simulink model "cs_robot"  (R2017b)
settings: Solver=FixedStepDiscrete  StartTime=0.0  StopTime=2  RelTol=1e-3  EnableMultiTasking=on
PreLoadFcn:
  | Ts=1e-6;
InitFcn:
  | Ts=1e-6;
undefined symbols (not defined in the file): DiscIntNeverNeededParam
libraries: powerlib x5, electricdrivelib x4
Description:
  | Copyright 2008-2017 The MathWorks, Inc.
settings Model: ExtModeAutoUpdateStatusClock=off  Creator=MathWorks  LastModifiedBy=Rafa
settings SolverCC: InsertRTBMode=Auto
settings DataIOCC: LimitDataPoints=on  SaveFormat=Array  SignalLoggingSaveFormat=ModelDataLogs  SignalLoggingName=sigsOut
settings OptimizationCC: ExpressionDepthLimit=2147483647  InitFltsAndDblsToZero=on  LifeSpan=inf
settings DebuggingCC: SaveWithParameterizedLinksMsg=none  UnderspecifiedInitializationDetection=Classic  MergeDetectMultiDrivingBlocksExec=none  CheckExecutionContextPreStartOutputMsg=on  CheckExecutionContextRuntimeOutputMsg=on  SignalResolutionControl=TryResolveAllWithWarning  MultiTaskDSMMsg=warning  MultiTaskCondExecSysMsg=none  FcnCallInpInsideContextMsg=warning  AllowSymbolicDim=off  StateNameClashWarn=warning  SFUnexpectedBacktrackingDiag=warning  SFNoUnconditionalDefaultTransitionDiag=warning  SFExecutionAtInitializationDiag=none
settings HardwareCC: ProdBitPerPointer=32  ProdBitPerSizeT=32  ProdBitPerPtrDiffT=32  ProdLargestAtomicFloat=None  ProdIntDivRoundTo=Undefined  ProdEndianess=Unspecified  ProdWordSize=32  ProdHWDeviceType=32-bit Generic  TargetBitPerPointer=64  TargetBitPerSizeT=64  TargetBitPerPtrDiffT=64  TargetLongLongMode=on  TargetIntDivRoundTo=Zero  TargetEndianess=LittleEndian  TargetWordSize=64  TargetHWDeviceType=MATLAB Host  ProdEqTarget=off
settings ModelReferenceCC: PropagateSignalLabelsOutOfModel=off
settings CodeAppCC: StateflowObjectComments=on
settings GRTTargetCC: TargetFcnLib=ansi_tfl_tmw.mat  TargetLangStandard=C89/C90 (ANSI)  GeneratePreprocessorConditionals=Disable all  CombineOutputUpdateFcns=off  GRTInterface=on
settings ConfigComp: CovMetricSettings=dw  CovHtmlReporting=on  CovSaveCumulativeToWorkspaceVar=on  CovSaveSingleToWorkspaceVar=on  CovExternalEMLEnable=off  CovSFcnEnable=off
settings SimscapeCC: SimscapeNormalizeSystem=off

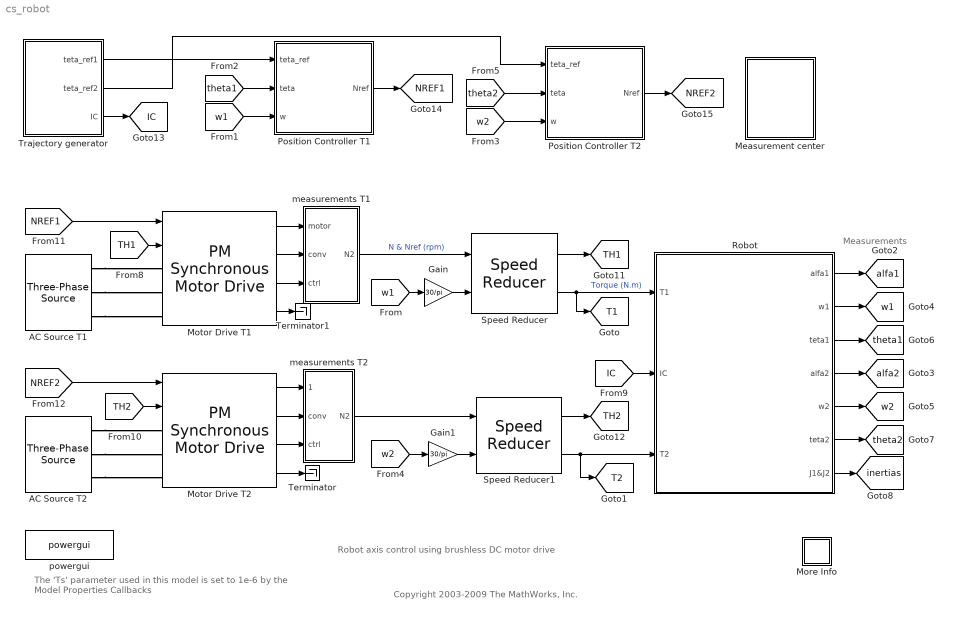
== system cs_robot ==
  note: Robot axis control using brushless DC motor drive
  note: The 'Ts' parameter used in this model
      | is set to 1e-6  by the Model Properties Callbacks
  note: Measurements
  note: Copyright 2003-2009 The MathWorks, Inc.
  AC Source T1 : powerlib/Electrical Sources/Three-Phase Source  InternalConnection=Yg  VoltagePhases=off  Voltage=220  PhaseAngle=0  Voltage_phases=[25e3 25e3 25e3]/sqrt(3)  PhaseAngles_phases=[0 -120 +120]  Frequency=60  NonIdealSource=on  SpecifyImpedance=off  Resistance=0.1  Inductance=0.1e-3  ShortCircuitLevel=0  BaseVoltage=0  XRratio=0  BusType=swing  Pref=0  Qref=0  Prefabc=0  Qrefabc=0  Qmin=-inf  Qmax=inf
  AC Source T2 : powerlib/Electrical Sources/Three-Phase Source  InternalConnection=Yg  VoltagePhases=off  Voltage=220  PhaseAngle=0  Voltage_phases=[25e3 25e3 25e3]/sqrt(3)  PhaseAngles_phases=[0 -120 +120]  Frequency=60  NonIdealSource=on  SpecifyImpedance=off  Resistance=0.1  Inductance=0.1e-3  ShortCircuitLevel=0  BaseVoltage=0  XRratio=0  BusType=swing  Pref=0  Qref=0  Prefabc=0  Qrefabc=0  Qmin=-inf  Qmax=inf
  Gain : Gain  Gain=30/pi  SaturateOnIntegerOverflow=on  OutDataTypeStr=Inherit: Same as input  ParamDataTypeStr=Inherit: Same as input
  Gain1 : Gain  Gain=30/pi  SaturateOnIntegerOverflow=on  OutDataTypeStr=Inherit: Same as input  ParamDataTypeStr=Inherit: Same as input
  Measurement center : Subsystem
  More Info : Subsystem
      settings: OpenFcn="docsearch('\"Robot axis control using brushless DC motor drive\"')"
      mask Display: disp('?')
  Motor Drive T1 : electricdrivelib/AC drives/PM Synchronous Motor Drive  Rs=0.2  Lls=8.5e-3  Lms=8.5e-3  MachineConstant=Flux linkage established by magnets (V.s)  FluxCst=0.175  VoltageCst=126.966  TorqueCst=1.05  ia=0  ib=0  J=0.01  Friction=0.005  p=4  wm=0  thetam=0  Rsnb_rec=10e3  Csnb_rec=20e-9  Ron_rec=1e-3  Vf_rec=1.3  cap_bus=2000e-6  Rbrake=8  fbrake=4000  activationVoltage=320  shutdownVoltage=310  sourceFrequency=60  deviceType=IGBT / Diodes  Ron_inv=1e-3  Vf_inv=0.8  Vfd_inv=0.8  Tf=1e-6  Tt=2e-6  Tf_GTO=0  Tt_GTO=0  Rsnb_inv=5000  Csnb_inv=inf  regulationType=Speed regulation  Acc=5000  Dec=-5000  kp_sc=0.5  ki_sc=10  fc_sc=1000  Tsc=140e-6  Tmin=-17.8*1.5  Tmax=17.8*1.5  modulationType=Hysteresis  h=0.1  kp_Id=200  ki_Id=1000  kp_Iq=200  ki_Iq=1000  fc_bus=50  car_freq=20000  freq_max=20e3  Tvect=20e-6  baseSampleTime=1e-06  outputBusMode=Multiple output buses  busLabels=off  MechanicalLoad=Torque Tm  modelDetailLevel=Detailed  driveType=AC6  AverageValue=off
      link override VECT: machineConstant=Flux linkage established by magnets (V.s)
      settings: SourceProductName=Simscape Power Systems  SourceProductBaseCode=PS
  Motor Drive T2 : electricdrivelib/AC drives/PM Synchronous Motor Drive  Rs=0.2  Lls=8.5e-3  Lms=8.5e-3  MachineConstant=Flux linkage established by magnets (V.s)  FluxCst=0.175  VoltageCst=126.966  TorqueCst=1.05  ia=0  ib=0  J=0.01  Friction=0.005  p=4  wm=0  thetam=0  Rsnb_rec=10e3  Csnb_rec=20e-9  Ron_rec=1e-3  Vf_rec=1.3  cap_bus=2000e-6  Rbrake=8  fbrake=4000  activationVoltage=320  shutdownVoltage=310  sourceFrequency=60  deviceType=IGBT / Diodes  Ron_inv=1e-3  Vf_inv=0.8  Vfd_inv=0.8  Tf=1e-6  Tt=2e-6  Tf_GTO=0  Tt_GTO=0  Rsnb_inv=5000  Csnb_inv=inf  regulationType=Speed regulation  Acc=5000  Dec=-5000  kp_sc=0.5  ki_sc=10  fc_sc=1000  Tsc=140e-6  Tmin=-17.8*1.5  Tmax=17.8*1.5  modulationType=Hysteresis  h=0.1  kp_Id=200  ki_Id=1000  kp_Iq=200  ki_Iq=1000  fc_bus=50  car_freq=20000  freq_max=20e3  Tvect=20e-6  baseSampleTime=1e-06  outputBusMode=Multiple output buses  busLabels=off  MechanicalLoad=Torque Tm  modelDetailLevel=Detailed  driveType=AC6  AverageValue=off
      link override VECT: machineConstant=Flux linkage established by magnets (V.s)
      settings: SourceProductName=Simscape Power Systems  SourceProductBaseCode=PS
  Position Controller T1 : Subsystem  mask{Kp=32000, Kd=400}
      mask prompts: Kp "Proportional gain"; Kd "Derivative gain"
  Position Controller T2 : Subsystem  mask{Kp=32000, Kd=400}
      mask prompts: Kp "Proportional gain"; Kd "Derivative gain"
  Robot : Subsystem
      mask Display:
      | image(imread('robot_5.bmp'))
      | port_label('output', 1, 'alfa1')
      | port_label('output', 2, 'w1')
      | port_label('output', 3, 'teta1')
      | port_label('input', 1, 'T1')
      | port_label('input', 2, 'IC')
      | port_label('output', 4, 'alfa2')
      | port_label('output', 5, 'w2')
      | port_label('output', 6, 'teta2')
      | port_label('input', 3, 'T2')
      | port_label('output', 7, 'J1_J2')
  Speed Reducer : electricdrivelib/Shafts and speed reducers/Speed Reducer  PresetModel=No  i=130  Jrdh=0.001  eff=1  Ksh=17190  Bsh=600  Ksl=17190*100  Bsl=600*300
      settings: SourceProductName=Simscape Power Systems  SourceProductBaseCode=PS
  Speed Reducer1 : electricdrivelib/Shafts and speed reducers/Speed Reducer  PresetModel=No  i=100  Jrdh=0.001  eff=1  Ksh=17190  Bsh=600  Ksl=17190*100  Bsl=600*300
      settings: SourceProductName=Simscape Power Systems  SourceProductBaseCode=PS
  Terminator : Terminator
  Terminator1 : Terminator
  Trajectory generator : Subsystem  mask{posini=[-30 -45], posfin=[30 45], tfin=1.5}
      mask prompts: posini "Initial positions [teta1 teta2] (degree)"; posfin "Final position [teta1 teta2] (degree)"; tfin "Final time (second)"
      mask init:
      | posini=posini*pi/180;
      | posfin=posfin*pi/180;
      | tetaini1=posini(1);
      | tetaini2=posini(2);
      | tetafin1=posfin(1);
      | tetafin2=posfin(2);
  measurements T1 : Subsystem
  measurements T2 : Subsystem
  powergui : powerlib/powergui  Priority=2  SimulationMode=Discrete  SampleTime=Ts  frequency=60  Iterations=50  frequencyindice=60  Pbase=100e6  ErrMax=1e-4  UnitsV=kV  UnitsW=MW  buscounter=0  FunctionMessages=off  echomessages=off  EnableUseOfTLC=off  CurrentSourceSwitches=off  DisableSnubberDevices=off  DisableRonSwitches=off  DisableVfSwitches=off  DisplayEquations=off  SolverType=Tustin  Interpol=off  ExternalGateDelay=off  methode=off  Ts=0  x0status=blocks  SPID=off  SwTol=0  HookPort=off  RestoreLinks=warning  ResistiveCurrentMeasurement=off  Frange=[0:2:500]  Ylog=off  Xlog=on  ShowGrid=off  save=off  variable=ZData  structure=0  ZoomFFT=on  StartTime=0.0  cycles=1  DisplayStyle=1  fundamental=60  FreqAxis=off  MaxFrequency=1000  frequencyindicesteady=1  RmsSteady=1  display=off
  tag scope: IC=global, NREF1=global, NREF2=global, T1=global, T2=global, TH1=global, TH2=global, alfa1=global, alfa2=global, inertias=global, theta1=global, theta2=global, w1=global, w2=global
  wires:
  Motor Drive T1/1 -> measurements T1/1(motor)
  Motor Drive T1/2 -> measurements T1/2(conv)
  Motor Drive T1/3 -> measurements T1/3(ctrl)
  Speed Reducer/2 -> Robot/1(T1), [T1]  "Torque (N.m)"
  Gain/1 -> Speed Reducer/2
  Motor Drive T2/1 -> measurements T2/1(motor)
  Motor Drive T2/2 -> measurements T2/2(conv)
  Motor Drive T2/3 -> measurements T2/3(ctrl)
  Robot/2(w1) -> [w1]
  Robot/3(teta1) -> [theta1]
  Speed Reducer1/2 -> Robot/3(T2), [T2]
  Gain1/1 -> Speed Reducer1/2
  Robot/6(teta2) -> [theta2]
  Speed Reducer/1 -> [TH1]
  Robot/1(alfa1) -> [alfa1]
  Robot/4(alfa2) -> [alfa2]
  Robot/7(J1&J2) -> [inertias]
  [w1] -> Gain/1
  [w1] -> Position Controller T1/3(w)
  [theta1] -> Position Controller T1/2(teta)
  [w2] -> Position Controller T2/3(w)
  [w2] -> Gain1/1
  Robot/5(w2) -> [w2]
  [theta2] -> Position Controller T2/2(teta)
  Trajectory generator/1(teta_ref1) -> Position Controller T1/1(teta_ref)
  Trajectory generator/2(teta_ref2) -> Position Controller T2/1(teta_ref)
  [TH1] -> Motor Drive T1/2
  Speed Reducer1/1 -> [TH2]
  [IC] -> Robot/2(IC)
  Trajectory generator/3(IC) -> [IC]
  [TH2] -> Motor Drive T2/2
  Position Controller T1/1(Nref) -> [NREF1]
  Position Controller T2/1(Nref) -> [NREF2]
  [NREF1] -> Motor Drive T1/1
  [NREF2] -> Motor Drive T2/1
  Motor Drive T2/4 -> Terminator/1
  Motor Drive T1/4 -> Terminator1/1
  measurements T1/1(N2) -> Speed Reducer/1  "N & Nref (rpm)"
  measurements T2/1(N2) -> Speed Reducer1/1
  connections:
  AC Source T1/RConn1 -- Motor Drive T1/LConn1
  AC Source T1/RConn2 -- Motor Drive T1/LConn2
  AC Source T1/RConn3 -- Motor Drive T1/LConn3
  AC Source T2/RConn1 -- Motor Drive T2/LConn1
  AC Source T2/RConn2 -- Motor Drive T2/LConn2
  AC Source T2/RConn3 -- Motor Drive T2/LConn3

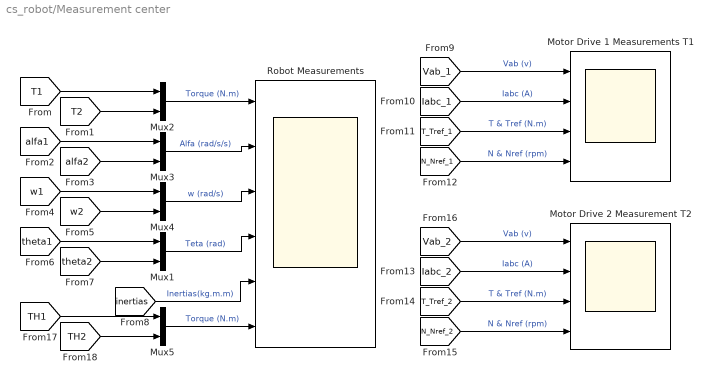
== system cs_robot/Measurement center ==
  Motor Drive 1 Measurements T1 : Scope  NumInputPorts=4
  Motor Drive 2 Measurement T2 : Scope  NumInputPorts=4
  Mux{1..5} (5 alike) : Mux  Inputs=2
  Robot Measurements : Scope  NumInputPorts=6
  wires:
  Mux1/1 -> Robot Measurements/4  "Teta (rad)"
  Mux2/1 -> Robot Measurements/1  "Torque (N.m)"
  Mux3/1 -> Robot Measurements/2  "Alfa (rad/s/s)"
  Mux4/1 -> Robot Measurements/3  "w (rad/s)"
  [T1] -> Mux2/1
  [T2] -> Mux2/2
  [alfa1] -> Mux3/1
  [alfa2] -> Mux3/2
  [w1] -> Mux4/1
  [w2] -> Mux4/2
  [theta1] -> Mux1/1
  [theta2] -> Mux1/2
  [inertias] -> Robot Measurements/5  "Inertias(kg.m.m)"
  [Vab_1] -> Motor Drive 1 Measurements T1/1  "Vab (v)"
  [Iabc_1] -> Motor Drive 1 Measurements T1/2  "Iabc (A)"
  [T_Tref_1] -> Motor Drive 1 Measurements T1/3  "T & Tref (N.m)"
  [N_Nref_1] -> Motor Drive 1 Measurements T1/4  "N & Nref (rpm)"
  [Vab_2] -> Motor Drive 2 Measurement T2/1  "Vab (v)"
  [Iabc_2] -> Motor Drive 2 Measurement T2/2  "Iabc (A)"
  [T_Tref_2] -> Motor Drive 2 Measurement T2/3  "T & Tref (N.m)"
  [N_Nref_2] -> Motor Drive 2 Measurement T2/4  "N & Nref (rpm)"
  [TH2] -> Mux5/2
  [TH1] -> Mux5/1
  Mux5/1 -> Robot Measurements/6  "Torque (N.m)"

== system cs_robot/More Info ==

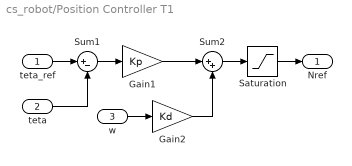
== system cs_robot/Position Controller T1 ==
  teta_ref : Inport
  teta : Inport  Port=2
  w : Inport  Port=3
  Gain1 : Gain  Gain=Kp  SaturateOnIntegerOverflow=on  OutDataTypeStr=Inherit: Same as input  ParamDataTypeStr=Inherit: Same as input
  Gain2 : Gain  Gain=Kd  SaturateOnIntegerOverflow=on  OutDataTypeStr=Inherit: Same as input  ParamDataTypeStr=Inherit: Same as input
  Saturation : Saturate  UpperLimit=2200  LowerLimit=-2200
  Sum1 : Sum  Inputs=|+-  SaturateOnIntegerOverflow=on
  Sum2 : Sum  Inputs=|++  SaturateOnIntegerOverflow=on
  Nref : Outport
  wires:
  Sum1/1 -> Gain1/1
  Gain1/1 -> Sum2/1
  Gain2/1 -> Sum2/2
  Sum2/1 -> Saturation/1
  Saturation/1 -> Nref/1
  teta_ref/1 -> Sum1/1
  teta/1 -> Sum1/2
  w/1 -> Gain2/1

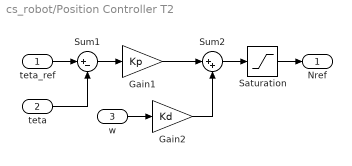
== system cs_robot/Position Controller T2 ==
  teta_ref : Inport
  teta : Inport  Port=2
  w : Inport  Port=3
  Gain1 : Gain  Gain=Kp  SaturateOnIntegerOverflow=on  OutDataTypeStr=Inherit: Same as input  ParamDataTypeStr=Inherit: Same as input
  Gain2 : Gain  Gain=Kd  SaturateOnIntegerOverflow=on  OutDataTypeStr=Inherit: Same as input  ParamDataTypeStr=Inherit: Same as input
  Saturation : Saturate  UpperLimit=2200  LowerLimit=-2200
  Sum1 : Sum  Inputs=|+-  SaturateOnIntegerOverflow=on
  Sum2 : Sum  Inputs=|++  SaturateOnIntegerOverflow=on
  Nref : Outport
  wires:
  w/1 -> Gain2/1
  teta/1 -> Sum1/2
  teta_ref/1 -> Sum1/1
  Saturation/1 -> Nref/1
  Sum2/1 -> Saturation/1
  Gain2/1 -> Sum2/2
  Gain1/1 -> Sum2/1
  Sum1/1 -> Gain1/1

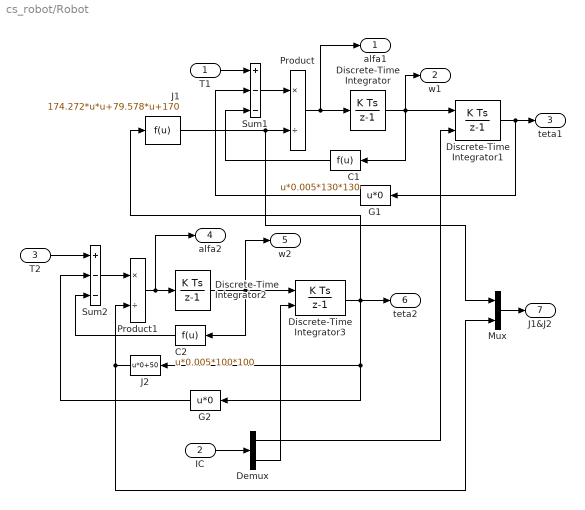
== system cs_robot/Robot ==
  T1 : Inport
  IC : Inport  Port=2
  T2 : Inport  Port=3
  C1 : Fcn  Expr=u*0.005*130*130
  C2 : Fcn  Expr=u*0.005*100*100
  Demux : Demux  Outputs=2
  Discrete-Time Integrator : DiscreteIntegrator  SampleTime=Ts  ICPrevOutput=DiscIntNeverNeededParam  ICPrevScaledInput=DiscIntNeverNeededParam
  Discrete-Time Integrator1 : DiscreteIntegrator  InitialConditionSource=external  SampleTime=Ts  ICPrevOutput=DiscIntNeverNeededParam  ICPrevScaledInput=DiscIntNeverNeededParam
  Discrete-Time Integrator2 : DiscreteIntegrator  SampleTime=Ts  ICPrevOutput=DiscIntNeverNeededParam  ICPrevScaledInput=DiscIntNeverNeededParam
  Discrete-Time Integrator3 : DiscreteIntegrator  InitialConditionSource=external  SampleTime=Ts  ICPrevOutput=DiscIntNeverNeededParam  ICPrevScaledInput=DiscIntNeverNeededParam
  G1 : Fcn  Expr=u*0
  G2 : Fcn  Expr=u*0
  J1 : Fcn  Expr=174.272*u*u+79.578*u+170
  J2 : Fcn  Expr=u*0+50
  Mux : Mux  Inputs=2
  Product : Product  Inputs=*/  SaturateOnIntegerOverflow=on  OutDataTypeStr=Inherit: Same as first input
  Product1 : Product  Inputs=*/  SaturateOnIntegerOverflow=on  OutDataTypeStr=Inherit: Same as first input
  Sum1 : Sum  Inputs=+--  SaturateOnIntegerOverflow=on
  Sum2 : Sum  Inputs=+--  SaturateOnIntegerOverflow=on
  alfa1 : Outport
  w1 : Outport  Port=2
  teta1 : Outport  Port=3
  alfa2 : Outport  Port=4
  w2 : Outport  Port=5
  teta2 : Outport  Port=6
  J1&J2 : Outport  Port=7
  wires:
  Product/1 -> Discrete-Time Integrator/1, alfa1/1
  Discrete-Time Integrator/1 -> Discrete-Time Integrator1/1, w1/1, C1/1
  T1/1 -> Sum1/1
  Discrete-Time Integrator1/1 -> teta1/1, G1/1
  Discrete-Time Integrator2/1 -> Discrete-Time Integrator3/1, C2/1, w2/1
  Product1/1 -> Discrete-Time Integrator2/1, alfa2/1
  Sum2/1 -> Product1/1
  C2/1 -> Sum2/3
  Discrete-Time Integrator3/1 -> G2/1, J2/1, teta2/1, J1/1
  G2/1 -> Sum2/2
  Sum1/1 -> Product/1
  C1/1 -> Sum1/3
  G1/1 -> Sum1/2
  J1/1 -> Product/2, Mux/1
  J2/1 -> Product1/2, Mux/2
  Demux/1 -> Discrete-Time Integrator1/2
  Demux/2 -> Discrete-Time Integrator3/2
  T2/1 -> Sum2/1
  IC/1 -> Demux/1
  Mux/1 -> J1&J2/1

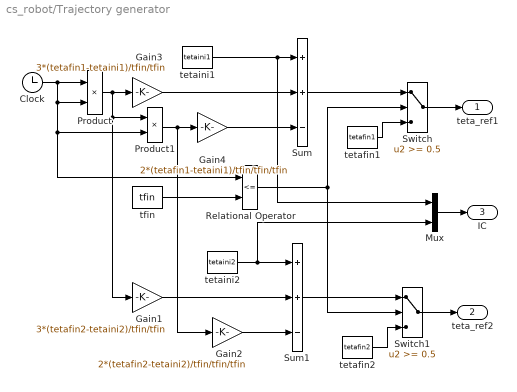
== system cs_robot/Trajectory generator ==
  Clock : Clock
  Gain1 : Gain  Gain=3*(tetafin2-tetaini2)/tfin/tfin  SaturateOnIntegerOverflow=on  OutDataTypeStr=Inherit: Same as input  ParamDataTypeStr=Inherit: Same as input
  Gain2 : Gain  Gain=2*(tetafin2-tetaini2)/tfin/tfin/tfin  SaturateOnIntegerOverflow=on  OutDataTypeStr=Inherit: Same as input  ParamDataTypeStr=Inherit: Same as input
  Gain3 : Gain  Gain=3*(tetafin1-tetaini1)/tfin/tfin  SaturateOnIntegerOverflow=on  OutDataTypeStr=Inherit: Same as input  ParamDataTypeStr=Inherit: Same as input
  Gain4 : Gain  Gain=2*(tetafin1-tetaini1)/tfin/tfin/tfin  SaturateOnIntegerOverflow=on  OutDataTypeStr=Inherit: Same as input  ParamDataTypeStr=Inherit: Same as input
  Mux : Mux  Inputs=2
  Product : Product  SaturateOnIntegerOverflow=on  OutDataTypeStr=Inherit: Same as first input
  Product1 : Product  SaturateOnIntegerOverflow=on  OutDataTypeStr=Inherit: Same as first input
  Relational Operator : RelationalOperator  Operator=<=  RndMeth=Nearest
  Sum : Sum  Inputs=++-  SaturateOnIntegerOverflow=on
  Sum1 : Sum  Inputs=++-  SaturateOnIntegerOverflow=on
  Switch : Switch  Threshold=0.5  SaturateOnIntegerOverflow=on
  Switch1 : Switch  Threshold=0.5  SaturateOnIntegerOverflow=on
  tetafin1 : Constant  Value=tetafin1
  tetafin2 : Constant  Value=tetafin2
  tetaini1 : Constant  Value=tetaini1
  tetaini2 : Constant  Value=tetaini2
  tfin : Constant  Value=tfin
  teta_ref1 : Outport
  teta_ref2 : Outport  Port=2
  IC : Outport  Port=3
  wires:
  Product1/1 -> Gain4/1, Gain2/1
  Gain4/1 -> Sum/3
  Gain3/1 -> Sum/2
  Product/1 -> Gain3/1, Product1/1, Gain1/1
  Clock/1 -> Product/2, Product1/2, Relational Operator/1, Product/1
  tetaini1/1 -> Sum/1, Mux/1
  Switch/1 -> teta_ref1/1
  Sum/1 -> Switch/1
  tetafin1/1 -> Switch/3
  Relational Operator/1 -> Switch/2, Switch1/2
  tfin/1 -> Relational Operator/2
  Gain2/1 -> Sum1/3
  Gain1/1 -> Sum1/2
  tetaini2/1 -> Sum1/1, Mux/2
  Sum1/1 -> Switch1/1
  tetafin2/1 -> Switch1/3
  Switch1/1 -> teta_ref2/1
  Mux/1 -> IC/1

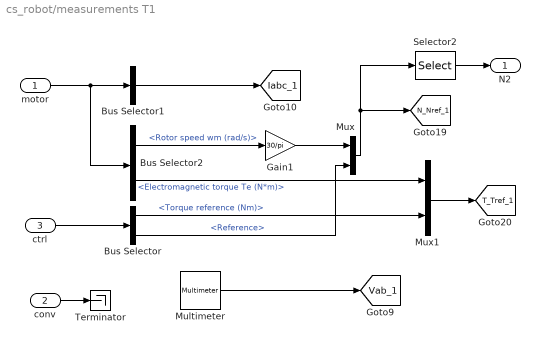
== system cs_robot/measurements T1 ==
  motor : Inport
  conv : Inport  Port=2
  ctrl : Inport  Port=3
  Bus Selector : BusSelector  OutputSignals=Torque reference (Nm),Reference
  Bus Selector1 : BusSelector  OutputSignals=Stator current is_a (A),Stator current is_b (A),Stator current is_c (A)  OutputAsBus=on
  Bus Selector2 : BusSelector  OutputSignals=Rotor speed wm (rad/s),Electromagnetic torque Te (N*m)
  Gain1 : Gain  Gain=30/pi  SaturateOnIntegerOverflow=on  OutDataTypeStr=Inherit: Same as input  ParamDataTypeStr=Inherit: Same as input
  Multimeter : powerlib/Measurements/Multimeter  PhasorSimulation=off  OutputType=Complex  sel=17  L=64  Gain=1  yselected={'Uab: Motor Drive T1/Three-phase diode rectifier'};  PSBOutputType=1  PSBequivalent=0  AxesSetting=[0,0.1,-100,100]  Display=0  SavedBlockNames=-11
  Mux : Mux  Inputs=2
  Mux1 : Mux  Inputs=2
  Selector2 : Selector  InputPortWidth=2  IndexOptions=Index vector (dialog)  Indices=1  OutputSizes=1
  Terminator : Terminator
  N2 : Outport
  tag scope: Iabc_1=global, N_Nref_1=global, T_Tref_1=global, Vab_1=global
  wires:
  Bus Selector2/2 -> Mux1/1  "<Electromagnetic torque Te (N*m)>"
  Gain1/1 -> Mux/1
  Bus Selector2/1 -> Gain1/1  "<Rotor speed wm (rad/s)>"
  Bus Selector1/1 -> [Iabc_1]
  Selector2/1 -> N2/1
  Multimeter/1 -> [Vab_1]
  motor/1 -> Bus Selector2/1, Bus Selector1/1
  ctrl/1 -> Bus Selector/1
  conv/1 -> Terminator/1
  Mux/1 -> Selector2/1, [N_Nref_1]
  Mux1/1 -> [T_Tref_1]
  Bus Selector/1 -> Mux1/2  "<Torque reference (Nm)>"
  Bus Selector/2 -> Mux/2  "<Reference>"

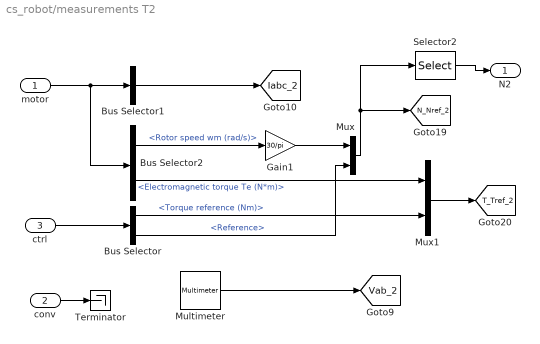
== system cs_robot/measurements T2 ==
  motor : Inport
  conv : Inport  Port=2
  ctrl : Inport  Port=3
  Bus Selector : BusSelector  OutputSignals=Torque reference (Nm),Reference
  Bus Selector1 : BusSelector  OutputSignals=Stator current is_a (A),Stator current is_b (A),Stator current is_c (A)  OutputAsBus=on
  Bus Selector2 : BusSelector  OutputSignals=Rotor speed wm (rad/s),Electromagnetic torque Te (N*m)
  Gain1 : Gain  Gain=30/pi  SaturateOnIntegerOverflow=on  OutDataTypeStr=Inherit: Same as input  ParamDataTypeStr=Inherit: Same as input
  Multimeter : powerlib/Measurements/Multimeter  PhasorSimulation=off  OutputType=Complex  sel=7  L=64  Gain=1  yselected={'Uab: Motor Drive T2/Three-phase diode rectifier'};  PSBOutputType=1  PSBequivalent=0  AxesSetting=[0,0.1,-100,100]  Display=0  SavedBlockNames=-11
  Mux : Mux  Inputs=2
  Mux1 : Mux  Inputs=2
  Selector2 : Selector  InputPortWidth=2  IndexOptions=Index vector (dialog)  Indices=1  OutputSizes=1
  Terminator : Terminator
  N2 : Outport
  tag scope: Iabc_2=global, N_Nref_2=global, T_Tref_2=global, Vab_2=global
  wires:
  Bus Selector/2 -> Mux/2  "<Reference>"
  Bus Selector/1 -> Mux1/2  "<Torque reference (Nm)>"
  Mux1/1 -> [T_Tref_2]
  Mux/1 -> [N_Nref_2], Selector2/1
  conv/1 -> Terminator/1
  ctrl/1 -> Bus Selector/1
  motor/1 -> Bus Selector1/1, Bus Selector2/1
  Multimeter/1 -> [Vab_2]
  Selector2/1 -> N2/1
  Bus Selector1/1 -> [Iabc_2]
  Bus Selector2/1 -> Gain1/1  "<Rotor speed wm (rad/s)>"
  Gain1/1 -> Mux/1
  Bus Selector2/2 -> Mux1/1  "<Electromagnetic torque Te (N*m)>"
